simulink model "curiser"  (R2023b)
settings: Solver=FixedStepDiscrete  StartTime=0.0  StopTime=10.0  RelTol=1e-3
settings Model: Creator=Beshary  LastModifiedBy=Beshary
settings OptimizationCC: DefaultParameterBehavior=Inlined  UseDivisionForNetSlopeComputation=on  GainParamInheritBuiltInType=on  UseFloatMulNetSlope=on  InlineInvariantSignals=on  PassReuseOutputArgsAs=Individual arguments  ZeroExternalMemoryAtStartup=off  ZeroInternalMemoryAtStartup=off  NoFixptDivByZeroProtection=on  EfficientFloat2IntCast=on  LifeSpan=1  OptimizeBlockOrder=speed  DifferentSizesBufferReuse=on  EfficientTunableParamExpr=on
settings DebuggingCC: ParameterTunabilityLossMsg=error  UnconnectedInputMsg=warning  UnconnectedOutputMsg=warning  UnconnectedLineMsg=warning
settings HardwareCC: ProdLongLongMode=on
settings ModelReferenceCC: EnableRefExpFcnMdlSchedulingChecks=on
settings SFSimCC: MATLABDynamicMemAlloc=off
settings RTWCC: Description=Embedded Coder  SystemTargetFile=ert.tlc  TemplateMakefile=ert_default_tmf  DLArmComputeVersion=19.05
settings CodeAppCC: ForceParamTrailComments=on  IgnoreCustomStorageClasses=off  OperatorAnnotations=on  SimulinkDataObjDesc=on  SFDataObjDesc=on  CustomSymbolStrGlobalVar=rt$N$M  CustomSymbolStrType=$N$M  CustomSymbolStrFcn=$N$M$F  CustomSymbolStrMacro=$N$M  InsertBlockDesc=on
settings ERTTargetCC: TargetLangStandard=C99 (ISO)  GenerateSampleERTMain=on  IncludeMdlTerminateFcn=off  CombineSignalStateStructs=on  SupportAbsoluteTime=off  SupportComplex=off  SupportNonInlinedSFcns=on  InlinedParameterPlacement=NonHierarchical  ERTCustomFileTemplate=example_file_process.tlc  ERTFilePackagingFormat=CompactWithDataFile

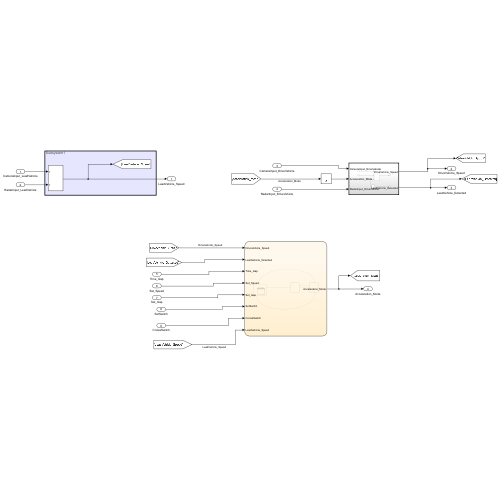
[thumbnail: Simulink's stored preview of the top-level diagram]
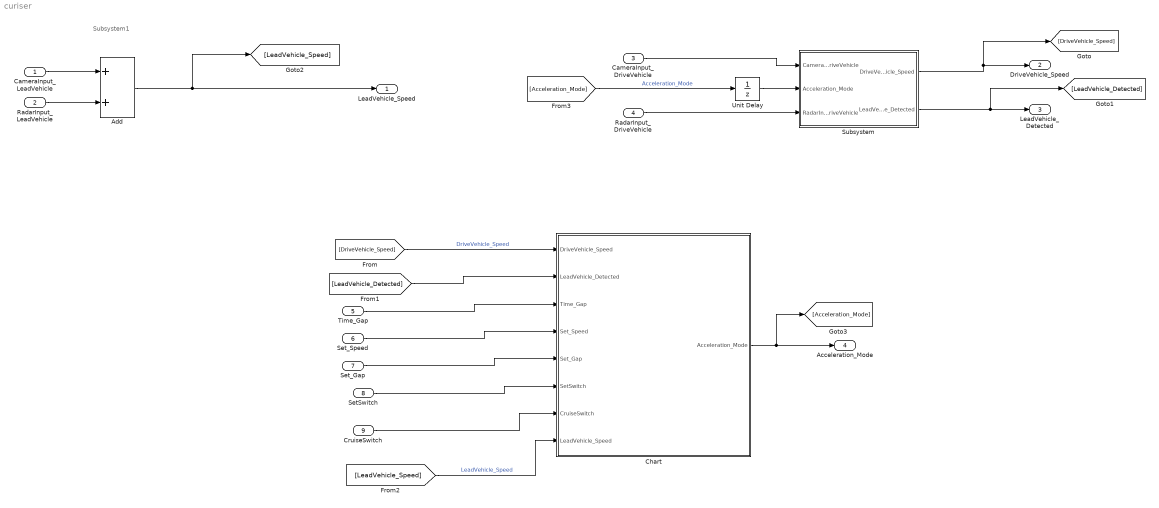
== system curiser ==
  note: Subsystem1
  CameraInput_LeadVehicle : Inport
  RadarInput_LeadVehicle : Inport  Port=2
  CameraInput_DriveVehicle : Inport  Port=3
  RadarInput_DriveVehicle : Inport  Port=4
  Time_Gap : Inport  Port=5
  Set_Speed : Inport  Port=6
  Set_Gap : Inport  Port=7
  SetSwitch : Inport  Port=8
  CruiseSwitch : Inport  Port=9
  Add : Sum
  Chart : Stateflow chart  TreatAsAtomicUnit=on
  Subsystem : Subsystem  TreatAsAtomicUnit=on
  Unit Delay : UnitDelay  SampleTime=-1  HasFrameUpgradeWarning=on
  LeadVehicle_Speed : Outport
  DriveVehicle_Speed : Outport  Port=2
  LeadVehicle_Detected : Outport  Port=3
  Acceleration_Mode : Outport  Port=4
  wires:
  CameraInput_DriveVehicle/1 -> Subsystem/1(CameraInput_DriveVehicle)
  [Acceleration_Mode] -> Unit Delay/1  "Acceleration_Mode"
  RadarInput_DriveVehicle/1 -> Subsystem/3(RadarInput_DriveVehicle)
  Subsystem/1(DriveVehicle_Speed) -> [DriveVehicle_Speed], DriveVehicle_Speed/1
  Subsystem/2(LeadVehicle_Detected) -> [LeadVehicle_Detected], LeadVehicle_Detected/1
  Time_Gap/1 -> Chart/3(Time_Gap)
  Set_Speed/1 -> Chart/4(Set_Speed)
  Set_Gap/1 -> Chart/5(Set_Gap)
  SetSwitch/1 -> Chart/6(SetSwitch)
  CruiseSwitch/1 -> Chart/7(CruiseSwitch)
  [LeadVehicle_Detected] -> Chart/2(LeadVehicle_Detected)
  [DriveVehicle_Speed] -> Chart/1(DriveVehicle_Speed)  "DriveVehicle_Speed"
  [LeadVehicle_Speed] -> Chart/8(LeadVehicle_Speed)  "LeadVehicle_Speed"
  Chart/1(Acceleration_Mode) -> [Acceleration_Mode], Acceleration_Mode/1
  Unit Delay/1 -> Subsystem/2(Acceleration_Mode)
  Add/1 -> LeadVehicle_Speed/1, [LeadVehicle_Speed]
  CameraInput_LeadVehicle/1 -> Add/1
  RadarInput_LeadVehicle/1 -> Add/2

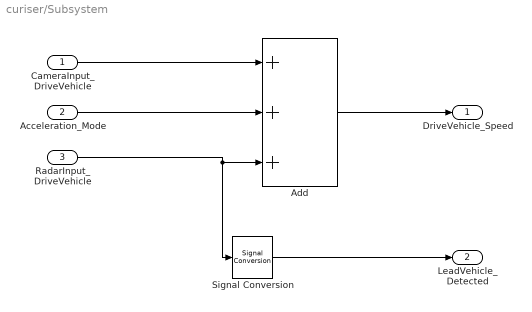
== system curiser/Subsystem ==
  CameraInput_DriveVehicle : Inport
  Acceleration_Mode : Inport  Port=2
  RadarInput_DriveVehicle : Inport  Port=3
  Add : Sum  Inputs=+++
  Signal Conversion : SignalConversion  OverrideOpt=off
  DriveVehicle_Speed : Outport
  LeadVehicle_Detected : Outport  Port=2
  wires:
  CameraInput_DriveVehicle/1 -> Add/1
  Acceleration_Mode/1 -> Add/2
  RadarInput_DriveVehicle/1 -> Signal Conversion/1, Add/3
  Add/1 -> DriveVehicle_Speed/1
  Signal Conversion/1 -> LeadVehicle_Detected/1

== stateflow chart curiser/Chart ==
  state OFF_Mode
    en:
    Acceleration_Mode=0;
  state STANDBY_Mode
    en:
    Acceleration_Mode==1;
  state ON_Mode
    state SubSystems
      state LeadVehicle_Speed_lessthan_Set_Speed
        en:
        Acceleration_Mode=4;
      state LeadVehicle_Detected_Follow
        en:
        Acceleration_Mode=2;
      state LeadVehicle_Not_Detected
        en:
        Acceleration_Mode =1;
      state LeadVehicle_Not_Detected_Resume
        en:
        Acceleration_Mode=1;
      state LeadVehicle_Detected_Resume
        en:Acceleration_Mode=3;
      state LeadVehicle_Speed_equal_Set_Speed
        en:
        Acceleration_Mode=5;
      (junction 71) -> LeadVehicle_Speed_lessthan_Set_Speed
      LeadVehicle_Speed_lessthan_Set_Speed -> (junction 66) [order 2] : [((LeadVehicle_Speed*1.25>=DriveVehicle_Speed) && (LeadVehicle_Speed * 0.75<=DriveVehicle_Speed)) && (DriveVehicle_Speed < Set_Speed) && ((Time_Gap<=1.25*Set_Gap) && (Time_Gap >=0.75*Set_Gap))]
      LeadVehicle_Detected_Follow -> LeadVehicle_Speed_lessthan_Set_Speed [order 2] : [(LeadVehicle_Detected == 1) && (LeadVehicle_Speed < Set_Speed) || (Time_Gap < Set_Gap)]
      LeadVehicle_Speed_lessthan_Set_Speed -> LeadVehicle_Not_Detected [order 1] : [(LeadVehicle_Detected == 0) && (DriveVehicle_Speed == Set_Speed)]
      LeadVehicle_Not_Detected -> LeadVehicle_Speed_lessthan_Set_Speed [order 2] : [(LeadVehicle_Detected == 1) && (LeadVehicle_Speed < Set_Speed) || (Time_Gap < Set_Gap)]
      (default) -> LeadVehicle_Detected_Follow
      LeadVehicle_Detected_Follow -> LeadVehicle_Not_Detected [order 1] : [LeadVehicle_Detected == 0]
      LeadVehicle_Detected_Resume -> LeadVehicle_Detected_Follow [order 1] : [(DriveVehicle_Speed == Set_Speed) && (LeadVehicle_Speed >= Set_Speed) && (Time_Gap >= Set_Gap)]
      LeadVehicle_Not_Detected -> LeadVehicle_Detected_Follow [order 1] : [(LeadVehicle_Detected==1) && (DriveVehicle_Speed == Set_Speed) && (LeadVehicle_Speed >= Set_Speed) && (Time_Gap >= Set_Gap)]
      (junction 66) -> LeadVehicle_Speed_equal_Set_Speed
      LeadVehicle_Speed_equal_Set_Speed -> (junction 71) [order 3] : [(LeadVehicle_Speed<Set_Speed) && (LeadVehicle_Speed<DriveVehicle_Speed) || (Time_Gap==0.75*Set_Gap)]
      LeadVehicle_Speed_equal_Set_Speed -> LeadVehicle_Not_Detected_Resume [order 1] : [(LeadVehicle_Detected == 0) || (DriveVehicle_Speed <= Set_Speed)]
      LeadVehicle_Detected_Resume -> LeadVehicle_Not_Detected_Resume [order 2] : [LeadVehicle_Detected==0]
      LeadVehicle_Speed_equal_Set_Speed -> LeadVehicle_Detected_Resume [order 2] : [(DriveVehicle_Speed < Set_Speed) && (LeadVehicle_Speed > DriveVehicle_Speed) || (Time_Gap >= Set_Gap)]
      LeadVehicle_Detected_Resume -> LeadVehicle_Speed_equal_Set_Speed [order 3] : [(DriveVehicle_Speed < Set_Speed) && (LeadVehicle_Speed > DriveVehicle_Speed) && (Time_Gap >= Set_Gap)]
  STANDBY_Mode -> ON_Mode [order 2] : [SetSwitch==1]
  (default) -> OFF_Mode
  STANDBY_Mode -> OFF_Mode [order 1] : [CruiseSwitch==0]
  ON_Mode -> OFF_Mode [order 1] : [CruiseSwitch==0]
  OFF_Mode -> STANDBY_Mode : [CruiseSwitch==1]
  ON_Mode -> STANDBY_Mode [order 2] : [SetSwitch==0]
  data: DriveVehicle_Speed input; LeadVehicle_Detected input; Time_Gap input; Set_Speed input; Set_Gap input; SetSwitch input; CruiseSwitch input; LeadVehicle_Speed input; Acceleration_Mode output
